simulink model "magball_linear"  (R2021b)
settings: Solver=VariableStepAuto  StartTime=0.0  StopTime=2.00  RelTol=1e-3
settings Model: Creator=rayya  LastModifiedBy=duzun
settings DebuggingCC: UnderSpecifiedDimensionMsg=warning

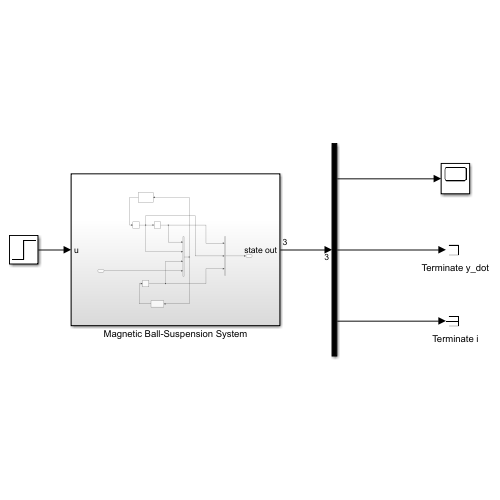
[thumbnail: Simulink's stored preview of the top-level diagram]
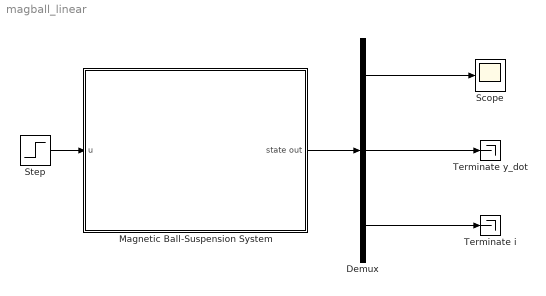
== system magball_linear ==
  Demux : Demux  Outputs=3
  Magnetic Ball-Suspension System : Subsystem
  Scope : Scope
  Step : Step  Time=0  SampleTime=0
  Terminate i : Terminator
  Terminate y_dot : Terminator
  wires:
  Demux/3 -> Terminate i/1
  Demux/2 -> Terminate y_dot/1
  Demux/1 -> Scope/1
  Step/1 -> Magnetic Ball-Suspension System/1(u)
  Magnetic Ball-Suspension System/1(state out) -> Demux/1

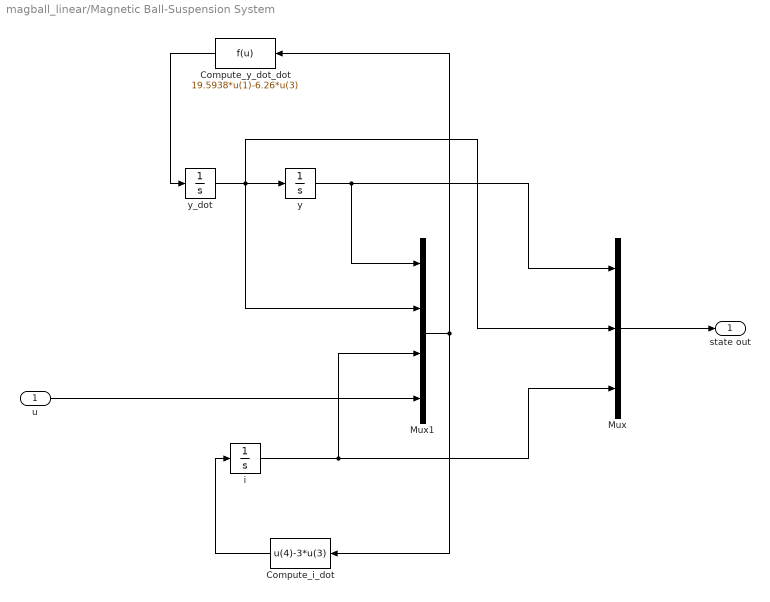
== system magball_linear/Magnetic Ball-Suspension System ==
  u : Inport
  Compute_i_dot : Fcn  Expr=u(4)-3*u(3)
  Compute_y_dot_dot : Fcn  Expr=19.5938*u(1)-6.26*u(3)
  Mux : Mux  Inputs=3
  Mux1 : Mux
  i : Integrator
  y : Integrator
  y_dot : Integrator
  state out : Outport
  wires:
  Compute_y_dot_dot/1 -> y_dot/1
  y/1 -> Mux1/1, Mux/1
  y_dot/1 -> Mux1/2, Mux/2, y/1
  i/1 -> Mux1/3, Mux/3
  u/1 -> Mux1/4
  Compute_i_dot/1 -> i/1
  Mux/1 -> state out/1
  Mux1/1 -> Compute_y_dot_dot/1, Compute_i_dot/1
